simulink model "lab3"  (R2015b)
settings: Solver=FixedStepDiscrete  StartTime=0.0  StopTime=10  FixedStep=0.03  RelTol=1e-3
undefined symbols (not defined in the file or in its folder): bias, DiscIntNeverNeededParam
libraries: RASPlib x2
settings Model: SimulationMode=external  ExtModeEnableFloating=off  ExtModeTrigDuration=4  ExtModeArchiveMode=auto  ExtModeArchiveFileName=w_x.mat  ExtModeArchiveDirName=/Users/kando/Documents/MATLAB/thesis/2016.12.29 RPI Mechatronics Labs/2.03  ExtModeWriteAllDataToWs=on  ExtModeLogAll=off  Creator=kando  LastModifiedBy=kando
settings DataIOCC: LimitDataPoints=off  SaveOutput=off  SignalLogging=off  DSMLogging=off  VisualizeSimOutput=off  SaveTime=off
settings OptimizationCC: OptimizeModelRefInitCode=on  LifeSpan=Inf  MaxStackSize=64
settings HardwareCC: ProdBitPerInt=16  ProdBitPerPointer=16  ProdLargestAtomicFloat=None  ProdWordSize=8  ProdHWDeviceType=Atmel->AVR
settings RTWCC: SystemTargetFile=ert.tlc  TemplateMakefile=ert_default_tmf  Description=Embedded Coder  Toolchain=Arduino AVR v1.6.1  BuildConfiguration=Faster Runs
settings CodeAppCC: IgnoreCustomStorageClasses=off
settings ERTTargetCC: SupportContinuousTime=on  SupportVariableSizeSignals=on  ExtMode=on  ExtModeMexFile=ext_serial_win32_comm_rtt  ExtModeMexArgs=1 '/dev/cu.usbmodem621' 115200

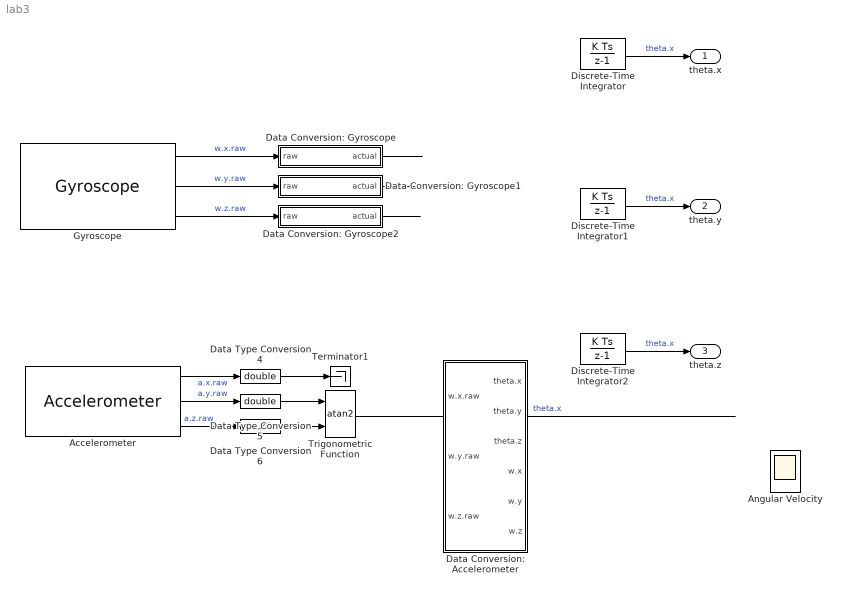
== system lab3 ==
  Accelerometer : RASPlib/Accelerometer  SimulateUsing=Code generation
  Angular Velocity : Scope
  Data Conversion: Accelerometer : Subsystem
  Data Conversion: Gyroscope : Subsystem
  Data Conversion: Gyroscope1 : Subsystem
  Data Conversion: Gyroscope2 : Subsystem
  Data Type Conversion4 : DataTypeConversion  OutDataTypeStr=double
  Data Type Conversion5 : DataTypeConversion  OutDataTypeStr=double
  Data Type Conversion6 : DataTypeConversion  OutDataTypeStr=double
  Discrete-Time Integrator : DiscreteIntegrator  ExternalReset=either  InitialConditionSetting=State (most efficient)  ICPrevOutput=DiscIntNeverNeededParam  ICPrevScaledInput=DiscIntNeverNeededParam
  Discrete-Time Integrator1 : DiscreteIntegrator  ExternalReset=either  InitialConditionSetting=State (most efficient)  ICPrevOutput=DiscIntNeverNeededParam  ICPrevScaledInput=DiscIntNeverNeededParam
  Discrete-Time Integrator2 : DiscreteIntegrator  ExternalReset=either  InitialConditionSetting=State (most efficient)  ICPrevOutput=DiscIntNeverNeededParam  ICPrevScaledInput=DiscIntNeverNeededParam
  Gyroscope : RASPlib/Gyroscope  DLPFmode=0
  Terminator1 : Terminator
  Trigonometric Function : Trigonometry  Operator=atan2
  theta.x : Outport
  theta.y : Outport  Port=2
  theta.z : Outport  Port=3
  wires:
  Gyroscope/1 -> Data Conversion: Gyroscope/1(raw)  "w.x.raw"
  Gyroscope/3 -> Data Conversion: Gyroscope2/1(raw)  "w.z.raw"
  Gyroscope/2 -> Data Conversion: Gyroscope1/1(raw)  "w.y.raw"
  Accelerometer/1 -> Data Type Conversion4/1  "a.x.raw"
  Accelerometer/3 -> Data Type Conversion6/1  "a.z.raw"
  Accelerometer/2 -> Data Type Conversion5/1  "a.y.raw"
  Trigonometric Function/1 -> ?  "theta.x"
  Data Type Conversion5/1 -> Trigonometric Function/1
  Data Type Conversion6/1 -> Trigonometric Function/2
  Data Type Conversion4/1 -> Terminator1/1
  Data Conversion: Gyroscope1/1(actual) -> ?
  Data Conversion: Gyroscope2/1(actual) -> ?
  Data Conversion: Gyroscope/1(actual) -> ?
  Discrete-Time Integrator/1 -> theta.x/1  "theta.x"
  ? -> Discrete-Time Integrator/2
  ? -> Discrete-Time Integrator/1  "w.x"
  Discrete-Time Integrator1/1 -> theta.y/1  "theta.x"
  ? -> Discrete-Time Integrator1/2
  ? -> Discrete-Time Integrator1/1  "w.y"
  Discrete-Time Integrator2/1 -> theta.z/1  "theta.x"
  ? -> Discrete-Time Integrator2/2
  ? -> Discrete-Time Integrator2/1  "w.z"

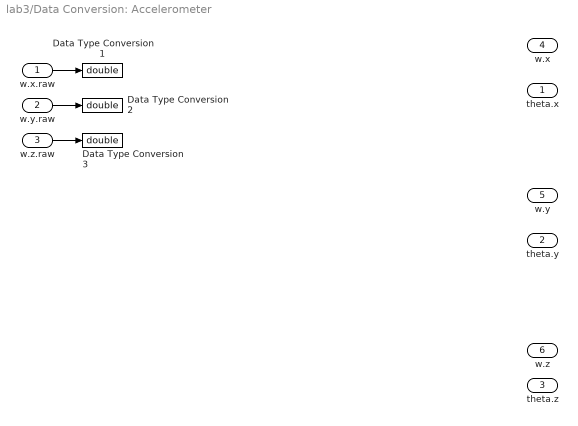
== system lab3/Data Conversion: Accelerometer ==
  w.x.raw : Inport
  w.y.raw : Inport  Port=2
  w.z.raw : Inport  Port=3
  Data Type Conversion1 : DataTypeConversion  OutDataTypeStr=double
  Data Type Conversion2 : DataTypeConversion  OutDataTypeStr=double
  Data Type Conversion3 : DataTypeConversion  OutDataTypeStr=double
  theta.x : Outport
  theta.y : Outport  Port=2
  theta.z : Outport  Port=3
  w.x : Outport  Port=4
  w.y : Outport  Port=5
  w.z : Outport  Port=6
  wires:
  w.z.raw/1 -> Data Type Conversion3/1
  w.y.raw/1 -> Data Type Conversion2/1
  w.x.raw/1 -> Data Type Conversion1/1

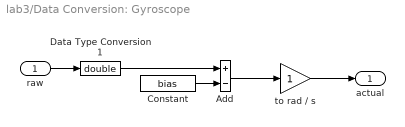
== system lab3/Data Conversion: Gyroscope ==
  raw : Inport
  " to rad / s" : Gain
  Add : Sum  Inputs=+-
  Constant : Constant  Value=bias
  Data Type Conversion1 : DataTypeConversion  OutDataTypeStr=double
  actual : Outport
  wires:
  Add/1 -> " to rad / s"/1
  Constant/1 -> Add/2
  raw/1 -> Data Type Conversion1/1
  Data Type Conversion1/1 -> Add/1
  " to rad / s"/1 -> actual/1

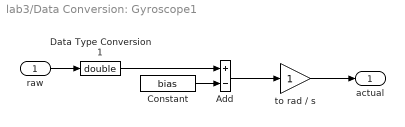
== system lab3/Data Conversion: Gyroscope1 ==
  raw : Inport
  " to rad / s" : Gain
  Add : Sum  Inputs=+-
  Constant : Constant  Value=bias
  Data Type Conversion1 : DataTypeConversion  OutDataTypeStr=double
  actual : Outport
  wires:
  " to rad / s"/1 -> actual/1
  Data Type Conversion1/1 -> Add/1
  raw/1 -> Data Type Conversion1/1
  Constant/1 -> Add/2
  Add/1 -> " to rad / s"/1

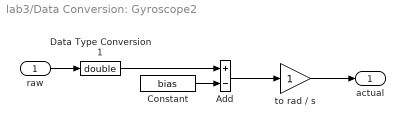
== system lab3/Data Conversion: Gyroscope2 ==
  raw : Inport
  " to rad / s" : Gain
  Add : Sum  Inputs=+-
  Constant : Constant  Value=bias
  Data Type Conversion1 : DataTypeConversion  OutDataTypeStr=double
  actual : Outport
  wires:
  Add/1 -> " to rad / s"/1
  Constant/1 -> Add/2
  raw/1 -> Data Type Conversion1/1
  Data Type Conversion1/1 -> Add/1
  " to rad / s"/1 -> actual/1
